simulink model "simu_lab1"  (R2022b)
settings: Solver=VariableStepAuto  StartTime=0.0  StopTime=1  MaxStep=1e-3  RelTol=1e-3
values from neighbouring files (symbols this model uses):
  result_k = mean(k_all)    [real_dataApprSimu_4_grapfs.m]
  result_Tm = mean(Tm_all)    [real_dataApprSimu_4_grapfs.m]
  U_pr = voltages(i)    [real_dataApprSimu_4_grapfs.m]
settings Model: Creator=serez  LastModifiedBy=serez

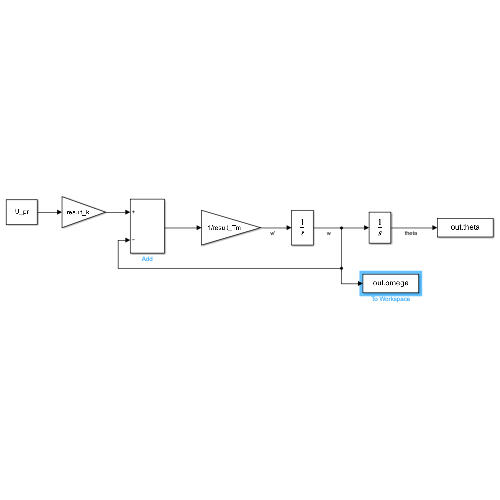
[thumbnail: Simulink's stored preview of the top-level diagram]
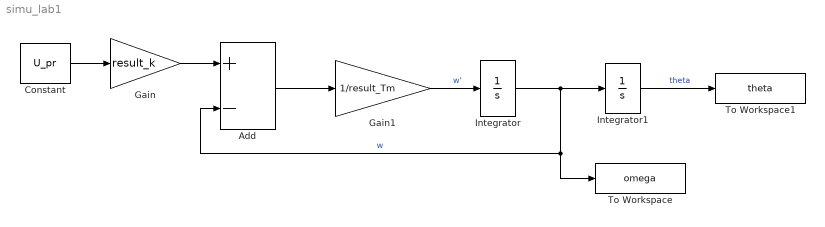
== system simu_lab1 ==
  Add : Sum  Inputs=+-
  Constant : Constant  Value=U_pr
  Gain : Gain  Gain=result_k
  Gain1 : Gain  Gain=1/result_Tm
  Integrator : Integrator
  Integrator1 : Integrator
  To Workspace : ToWorkspace  VariableName=omega  SaveFormat=Timeseries  SampleTime=-1
  To Workspace1 : ToWorkspace  VariableName=theta  SaveFormat=Timeseries  SampleTime=-1
  wires:
  Constant/1 -> Gain/1
  Gain/1 -> Add/1
  Add/1 -> Gain1/1
  Gain1/1 -> Integrator/1  "w'"
  Integrator/1 -> To Workspace/1, Add/2, Integrator1/1  "w"
  Integrator1/1 -> To Workspace1/1  "theta"
